simulink subsystem "DiffusivityScale"  (R2021b)
settings: Solver=VariableStepAuto  StartTime=0.0  StopTime=10.0  RelTol=1e-3
undefined symbols (not defined in the file): referenceXenonSaltDiffusivity
settings Model: Creator=Jiaqi  LastModifiedBy=Jiaqi

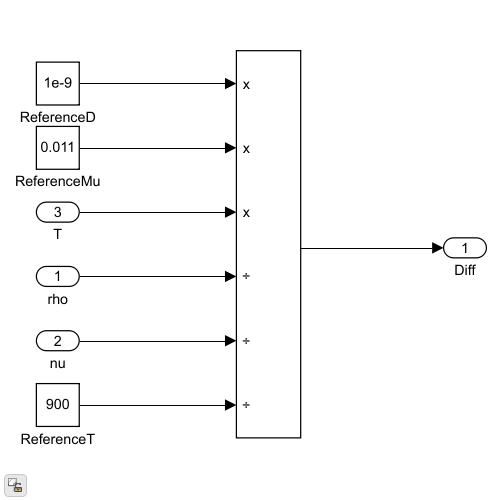
[thumbnail: Simulink's stored preview of the top-level diagram]
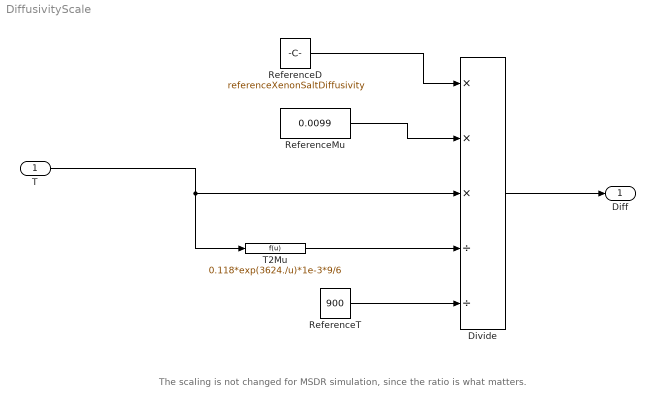
== system DiffusivityScale ==
  note: The scaling is not changed for MSDR simulation, since the ratio is what matters.
  T : Inport
  Divide : Product  Inputs=***//
  ReferenceD : Constant  Value=referenceXenonSaltDiffusivity
  ReferenceMu : Constant  Value=0.0099
  ReferenceT : Constant  Value=900
  T2Mu : Fcn  Expr=0.118*exp(3624./u)*1e-3*9/6
  Diff : Outport
  wires:
  ReferenceD/1 -> Divide/1
  ReferenceMu/1 -> Divide/2
  ReferenceT/1 -> Divide/5
  T/1 -> Divide/3, T2Mu/1
  Divide/1 -> Diff/1
  T2Mu/1 -> Divide/4
